simulink model "Controladoresplot"  (R2023b)
settings: Solver=ode1  StartTime=0.0  StopTime=70  FixedStep=1e-1  RelTol=1e-3  EnableMultiTasking=on
values from neighbouring files (symbols this model uses):
  C50_1 = 6.33    [P1.m]
  C50_2 = 6.76    [P2.m]
  C50_3 = 8.44    [P3.m]
  C50_4 = 6.44    [P4.m]
  Emax_1 = 94.1    [P1.m]
  Emax_2 = 86.0    (= 86)    [P2.m]
  Emax_3 = 80.7    [P3.m]
  Emax_4 = 102    [P4.m]
  gamma_1 = 2.24    [P1.m]
  gamma_2 = 4.29    [P2.m]
  gamma_3 = 4.10    (= 4.1)    [P3.m]
  gamma_4 = 2.18    [P4.m]
  k10_1 = Cl1_1 / V1    (= 0.38895787371)    [P1.m]
  k10_2 = Cl1_2 / V1    (= 0.37754352967)    [P2.m]
  k10_3 = Cl1_3 / V1    (= 0.386157411043)    [P3.m]
  k10_4 = Cl1_4 / V1    (= 0.323607493475)    [P4.m]
  k12_1 = Cl2_1 / V1    (= 0.375175644028)    [P1.m]
  k12_2 = Cl2_2 / V1    (= 0.397658079625)    [P2.m]
  k12_3 = Cl2_3 / V1    (= 0.44262295082)    [P3.m]
  k12_4 = Cl2_4 / V1    (= 0.318969555035)    [P4.m]
  k13_1 = Cl3_1 / V1    (= 0.195784543326)    [P1.m]
  k13_2 = Cl3_2 / V1    (= 0.195784543326)    [P2.m]
  k13_3 = Cl3_3 / V1    (= 0.195784543326)    [P3.m]
  k13_4 = Cl3_4 / V1    (= 0.195784543326)    [P4.m]
  k21_1 = Cl2_1/V2    (= 0.0667973147646)    [P1.m]
  k21_2 = Cl2_2/V2    (= 0.0664657298313)    [P2.m]
  k21_3 = Cl2_3/V2    (= 0.0659110723627)    [P3.m]
  k21_4 = Cl2_4/V2    (= 0.0678523389628)    [P4.m]
  k31_1 = Cl3_1/V3    (= 0.00351260504202)    [P1.m]
  k31_2 = Cl3_2/V3    (= 0.00351260504202)    [P2.m]
  k31_3 = Cl3_3/V3    (= 0.00351260504202)    [P3.m]
  k31_4 = Cl3_4/V3    (= 0.00351260504202)    [P4.m]
settings Model: Creator=Ana Gaby  LastModifiedBy=jeaze
settings SolverCC: AlgebraicLoopSolver=LineSearch
settings DataIOCC: LimitDataPoints=on  SaveFormat=Array  SignalLoggingSaveFormat=ModelDataLogs  ReturnWorkspaceOutputs=off
settings OptimizationCC: ExpressionDepthLimit=2147483647  LifeSpan=inf
settings DebuggingCC: UnderspecifiedInitializationDetection=Classic  MergeDetectMultiDrivingBlocksExec=none  SolverPrmCheckMsg=warning  FcnCallInpInsideContextMsg=warning  UnconnectedInputMsg=warning  UnconnectedOutputMsg=warning  UnconnectedLineMsg=warning  StateNameClashWarn=warning  SFUnexpectedBacktrackingDiag=warning  SFNoUnconditionalDefaultTransitionDiag=warning  SFExecutionAtInitializationDiag=none  ArithmeticOperatorsInVariantConditions=warning
settings HardwareCC: ProdBitPerPointer=32  ProdBitPerSizeT=32  ProdBitPerPtrDiffT=32  ProdLargestAtomicFloat=None  ProdIntDivRoundTo=Undefined  ProdEndianess=Unspecified  ProdWordSize=32  ProdHWDeviceType=32-bit Generic
settings ModelReferenceCC: EnableRefExpFcnMdlSchedulingChecks=on  PropagateSignalLabelsOutOfModel=off
settings SFSimCC: SimUseLocalCustomCode=off  SimParseCustomCode=off  CustomCodeUndefinedFunction=UseInterfaceOnly
settings RTWCC: RTWUseLocalCustomCode=off
settings CodeAppCC: StateflowObjectComments=on
settings GRTTargetCC: TargetLangStandard=C89/C90 (ANSI)  CombineOutputUpdateFcns=off  GRTInterface=on
settings ConfigComp: CovMetricSettings=dw  CovSaveCumulativeToWorkspaceVar=on  CovSaveSingleToWorkspaceVar=on  CovExternalEMLEnable=off

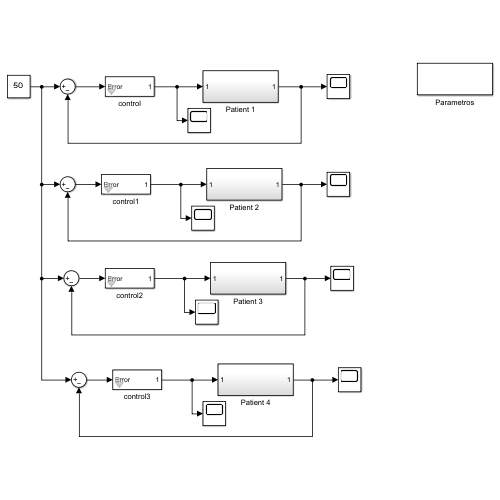
[thumbnail: Simulink's stored preview of the top-level diagram]
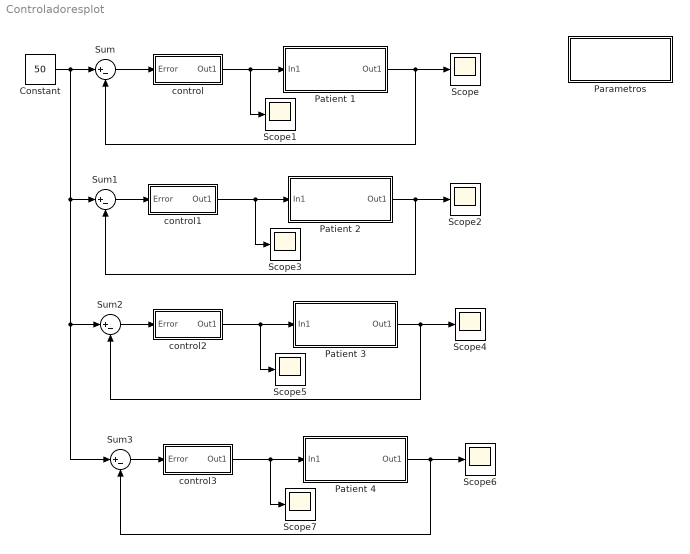
== system Controladoresplot ==
  Constant : Constant  Value=50
  Parametros : Subsystem
      settings: OpenFcn=|
      | P1
      | P2
      | P3
      | P4
  Patient 1 : Subsystem
  Patient 2 : Subsystem
  Patient 3 : Subsystem
  Patient 4 : Subsystem
  Scope{,1..7} (8 alike) : Scope
  Sum{,1..3} (4 alike) : Sum  Inputs=|+-
  control : Subsystem  mask{alfa=-100, Beta1=1}
  control1 : Subsystem  mask{alfa=-100, Beta1=1}
  control2 : Subsystem  mask{alfa=-100, Beta1=1}
  control3 : Subsystem  mask{alfa=-100, Beta1=1}
  wires:
  Patient 1/1(Out1) -> Scope/1, Sum/2
  control/1(Out1) -> Scope1/1, Patient 1/1(In1)
  Sum/1 -> control/1(Error)
  Constant/1 -> Sum/1, Sum1/1, Sum2/1, Sum3/1
  Patient 2/1(Out1) -> Scope2/1, Sum1/2
  control1/1(Out1) -> Patient 2/1(In1), Scope3/1
  Sum1/1 -> control1/1(Error)
  Patient 3/1(Out1) -> Scope4/1, Sum2/2
  control2/1(Out1) -> Patient 3/1(In1), Scope5/1
  Sum2/1 -> control2/1(Error)
  Patient 4/1(Out1) -> Scope6/1, Sum3/2
  control3/1(Out1) -> Patient 4/1(In1), Scope7/1
  Sum3/1 -> control3/1(Error)

== system Controladoresplot/Parametros ==

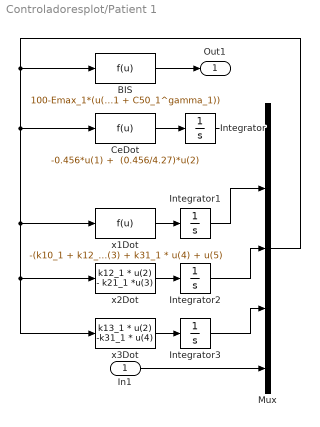
== system Controladoresplot/Patient 1 ==
  In1 : Inport
  BIS : Fcn  Expr=100-Emax_1*(u(1)^gamma_1/(u(1)^gamma_1 + C50_1^gamma_1))
  CeDot : Fcn  Expr="-0.456*u(1) +  (0.456/4.27)*u(2)"
  Integrator{,1..3} (4 alike) : Integrator
  Mux : Mux  Inputs=5
  x1Dot : Fcn  Expr=-(k10_1 + k12_1 + k13_1)*u(2) + k21_1 * u(3) + k31_1 * u(4) + u(5)
  x2Dot : Fcn  Expr=k12_1 * u(2) - k21_1 *u(3)
  x3Dot : Fcn  Expr=k13_1 * u(2) -k31_1 * u(4)
  Out1 : Outport  VectorParamsAs1DForOutWhenUnconnected=off
  wires:
  BIS/1 -> Out1/1
  CeDot/1 -> Integrator/1
  x1Dot/1 -> Integrator1/1
  x2Dot/1 -> Integrator2/1
  x3Dot/1 -> Integrator3/1
  Integrator/1 -> Mux/1
  Integrator1/1 -> Mux/2
  Integrator2/1 -> Mux/3
  Integrator3/1 -> Mux/4
  In1/1 -> Mux/5
  Mux/1 -> x3Dot/1, x2Dot/1, x1Dot/1, CeDot/1, BIS/1

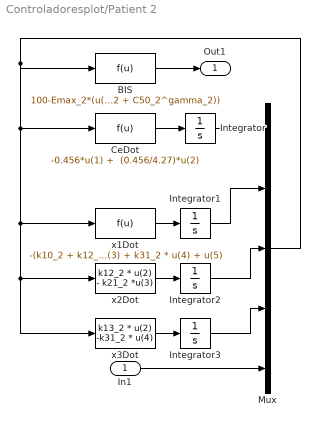
== system Controladoresplot/Patient 2 ==
  In1 : Inport
  BIS : Fcn  Expr=100-Emax_2*(u(1)^gamma_2/(u(1)^gamma_2 + C50_2^gamma_2))
  CeDot : Fcn  Expr="-0.456*u(1) +  (0.456/4.27)*u(2)"
  Integrator{,1..3} (4 alike) : Integrator
  Mux : Mux  Inputs=5
  x1Dot : Fcn  Expr=-(k10_2 + k12_2 + k13_2)*u(2) + k21_2 * u(3) + k31_2 * u(4) + u(5)
  x2Dot : Fcn  Expr=k12_2 * u(2) - k21_2 *u(3)
  x3Dot : Fcn  Expr=k13_2 * u(2) -k31_2 * u(4)
  Out1 : Outport  VectorParamsAs1DForOutWhenUnconnected=off
  wires:
  BIS/1 -> Out1/1
  CeDot/1 -> Integrator/1
  x1Dot/1 -> Integrator1/1
  x2Dot/1 -> Integrator2/1
  x3Dot/1 -> Integrator3/1
  Integrator/1 -> Mux/1
  Integrator1/1 -> Mux/2
  Integrator2/1 -> Mux/3
  Integrator3/1 -> Mux/4
  In1/1 -> Mux/5
  Mux/1 -> x3Dot/1, x2Dot/1, x1Dot/1, CeDot/1, BIS/1

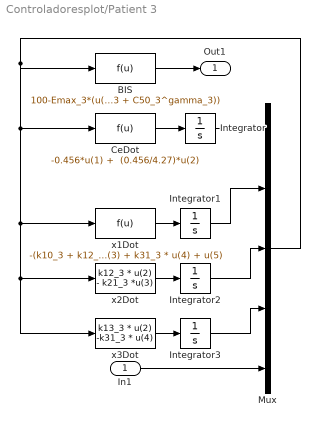
== system Controladoresplot/Patient 3 ==
  In1 : Inport
  BIS : Fcn  Expr=100-Emax_3*(u(1)^gamma_3/(u(1)^gamma_3 + C50_3^gamma_3))
  CeDot : Fcn  Expr="-0.456*u(1) +  (0.456/4.27)*u(2)"
  Integrator{,1..3} (4 alike) : Integrator
  Mux : Mux  Inputs=5
  x1Dot : Fcn  Expr=-(k10_3 + k12_3 + k13_3)*u(2) + k21_3 * u(3) + k31_3 * u(4) + u(5)
  x2Dot : Fcn  Expr=k12_3 * u(2) - k21_3 *u(3)
  x3Dot : Fcn  Expr=k13_3 * u(2) -k31_3 * u(4)
  Out1 : Outport  VectorParamsAs1DForOutWhenUnconnected=off
  wires:
  BIS/1 -> Out1/1
  CeDot/1 -> Integrator/1
  x1Dot/1 -> Integrator1/1
  x2Dot/1 -> Integrator2/1
  x3Dot/1 -> Integrator3/1
  Integrator/1 -> Mux/1
  Integrator1/1 -> Mux/2
  Integrator2/1 -> Mux/3
  Integrator3/1 -> Mux/4
  In1/1 -> Mux/5
  Mux/1 -> x3Dot/1, x2Dot/1, x1Dot/1, CeDot/1, BIS/1

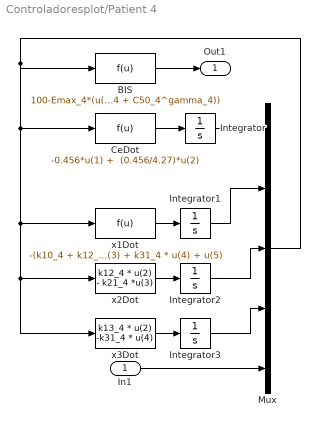
== system Controladoresplot/Patient 4 ==
  In1 : Inport
  BIS : Fcn  Expr=100-Emax_4*(u(1)^gamma_4/(u(1)^gamma_4 + C50_4^gamma_4))
  CeDot : Fcn  Expr="-0.456*u(1) +  (0.456/4.27)*u(2)"
  Integrator{,1..3} (4 alike) : Integrator
  Mux : Mux  Inputs=5
  x1Dot : Fcn  Expr=-(k10_4 + k12_4 + k13_4)*u(2) + k21_4 * u(3) + k31_4 * u(4) + u(5)
  x2Dot : Fcn  Expr=k12_4 * u(2) - k21_4 *u(3)
  x3Dot : Fcn  Expr=k13_4 * u(2) -k31_4 * u(4)
  Out1 : Outport  VectorParamsAs1DForOutWhenUnconnected=off
  wires:
  BIS/1 -> Out1/1
  CeDot/1 -> Integrator/1
  x1Dot/1 -> Integrator1/1
  x2Dot/1 -> Integrator2/1
  x3Dot/1 -> Integrator3/1
  Integrator/1 -> Mux/1
  Integrator1/1 -> Mux/2
  Integrator2/1 -> Mux/3
  Integrator3/1 -> Mux/4
  In1/1 -> Mux/5
  Mux/1 -> x3Dot/1, x2Dot/1, x1Dot/1, CeDot/1, BIS/1

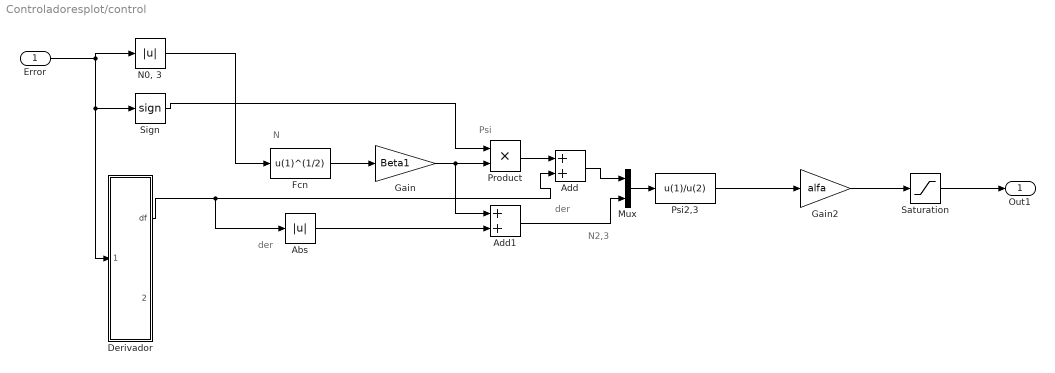
== system Controladoresplot/control ==
  note: Psi
  note: N
  note: der
  note: der
  note: N2,3
  Error : Inport
  Abs : Abs  SaturateOnIntegerOverflow=off
  Add : Sum
  Add1 : Sum
  Derivador : Subsystem
  Fcn : Fcn  Expr=u(1)^(1/2)
  Gain : Gain  Gain=Beta1
  Gain2 : Gain  Gain=alfa
  Mux : Mux  Inputs=2
  "N0, 3" : Abs  SaturateOnIntegerOverflow=off
  Product : Product  RndMeth=Zero
  Psi2,3 : Fcn  Expr=u(1)/u(2)
  Saturation : Saturate  UpperLimit=inf  LowerLimit=0
  Sign : Signum
  Out1 : Outport  VectorParamsAs1DForOutWhenUnconnected=off
  wires:
  Error/1 -> "N0, 3"/1, Sign/1, Derivador/1(In1)
  Fcn/1 -> Gain/1
  Gain/1 -> Product/2, Add1/1
  Product/1 -> Add/1
  Abs/1 -> Add1/2
  Mux/1 -> Psi2,3/1
  Add/1 -> Mux/1
  Add1/1 -> Mux/2
  "N0, 3"/1 -> Fcn/1
  Sign/1 -> Product/1
  Derivador/1(df) -> Abs/1, Add/2
  Gain2/1 -> Saturation/1
  Saturation/1 -> Out1/1
  Psi2,3/1 -> Gain2/1

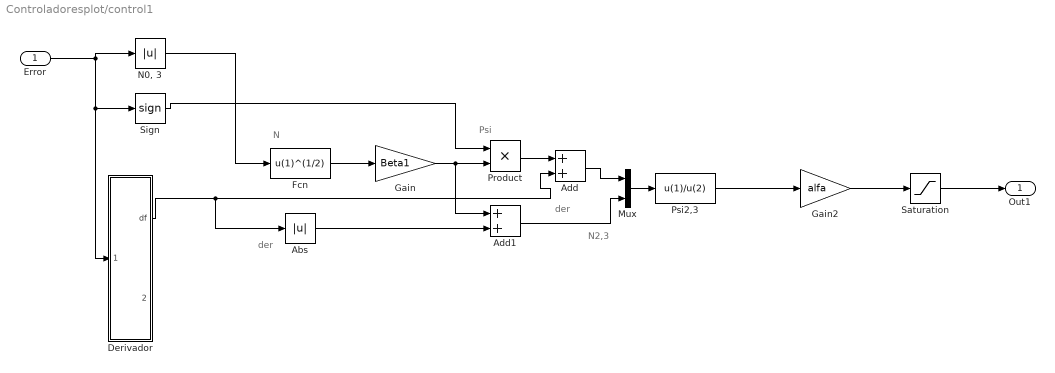
== system Controladoresplot/control1 ==
  note: Psi
  note: N
  note: der
  note: der
  note: N2,3
  Error : Inport
  Abs : Abs  SaturateOnIntegerOverflow=off
  Add : Sum
  Add1 : Sum
  Derivador : Subsystem
  Fcn : Fcn  Expr=u(1)^(1/2)
  Gain : Gain  Gain=Beta1
  Gain2 : Gain  Gain=alfa
  Mux : Mux  Inputs=2
  "N0, 3" : Abs  SaturateOnIntegerOverflow=off
  Product : Product  RndMeth=Zero
  Psi2,3 : Fcn  Expr=u(1)/u(2)
  Saturation : Saturate  UpperLimit=inf  LowerLimit=0
  Sign : Signum
  Out1 : Outport  VectorParamsAs1DForOutWhenUnconnected=off
  wires:
  Error/1 -> "N0, 3"/1, Sign/1, Derivador/1(In1)
  Fcn/1 -> Gain/1
  Gain/1 -> Product/2, Add1/1
  Product/1 -> Add/1
  Abs/1 -> Add1/2
  Mux/1 -> Psi2,3/1
  Add/1 -> Mux/1
  Add1/1 -> Mux/2
  "N0, 3"/1 -> Fcn/1
  Sign/1 -> Product/1
  Derivador/1(df) -> Abs/1, Add/2
  Gain2/1 -> Saturation/1
  Saturation/1 -> Out1/1
  Psi2,3/1 -> Gain2/1

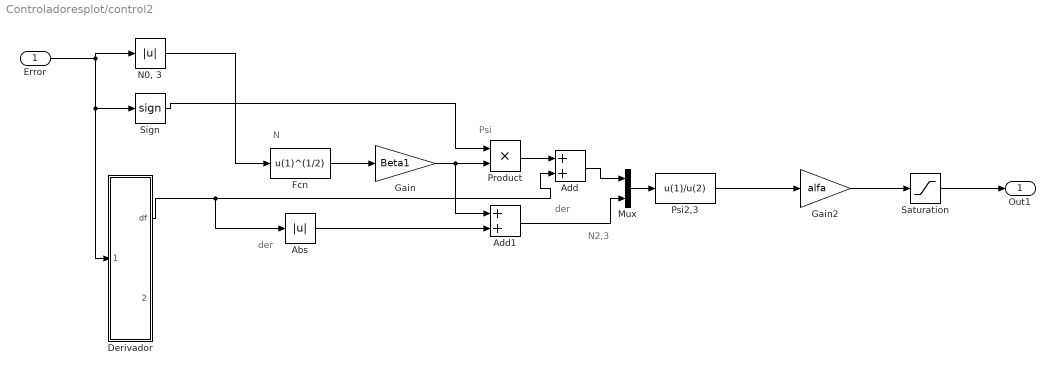
== system Controladoresplot/control2 ==
  note: Psi
  note: N
  note: der
  note: der
  note: N2,3
  Error : Inport
  Abs : Abs  SaturateOnIntegerOverflow=off
  Add : Sum
  Add1 : Sum
  Derivador : Subsystem
  Fcn : Fcn  Expr=u(1)^(1/2)
  Gain : Gain  Gain=Beta1
  Gain2 : Gain  Gain=alfa
  Mux : Mux  Inputs=2
  "N0, 3" : Abs  SaturateOnIntegerOverflow=off
  Product : Product  RndMeth=Zero
  Psi2,3 : Fcn  Expr=u(1)/u(2)
  Saturation : Saturate  UpperLimit=inf  LowerLimit=0
  Sign : Signum
  Out1 : Outport  VectorParamsAs1DForOutWhenUnconnected=off
  wires:
  Error/1 -> "N0, 3"/1, Sign/1, Derivador/1(In1)
  Fcn/1 -> Gain/1
  Gain/1 -> Product/2, Add1/1
  Product/1 -> Add/1
  Abs/1 -> Add1/2
  Mux/1 -> Psi2,3/1
  Add/1 -> Mux/1
  Add1/1 -> Mux/2
  "N0, 3"/1 -> Fcn/1
  Sign/1 -> Product/1
  Derivador/1(df) -> Abs/1, Add/2
  Gain2/1 -> Saturation/1
  Saturation/1 -> Out1/1
  Psi2,3/1 -> Gain2/1

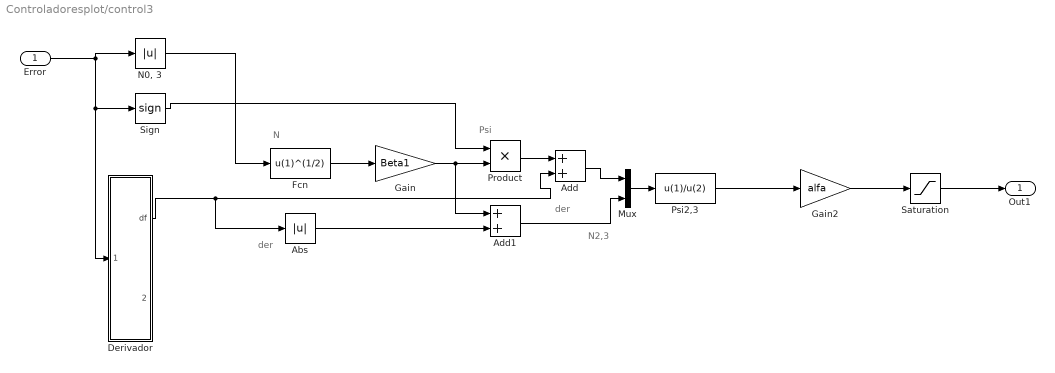
== system Controladoresplot/control3 ==
  note: Psi
  note: N
  note: der
  note: der
  note: N2,3
  Error : Inport
  Abs : Abs  SaturateOnIntegerOverflow=off
  Add : Sum
  Add1 : Sum
  Derivador : Subsystem
  Fcn : Fcn  Expr=u(1)^(1/2)
  Gain : Gain  Gain=Beta1
  Gain2 : Gain  Gain=alfa
  Mux : Mux  Inputs=2
  "N0, 3" : Abs  SaturateOnIntegerOverflow=off
  Product : Product  RndMeth=Zero
  Psi2,3 : Fcn  Expr=u(1)/u(2)
  Saturation : Saturate  UpperLimit=inf  LowerLimit=0
  Sign : Signum
  Out1 : Outport  VectorParamsAs1DForOutWhenUnconnected=off
  wires:
  Error/1 -> "N0, 3"/1, Sign/1, Derivador/1(In1)
  Fcn/1 -> Gain/1
  Gain/1 -> Product/2, Add1/1
  Product/1 -> Add/1
  Abs/1 -> Add1/2
  Mux/1 -> Psi2,3/1
  Add/1 -> Mux/1
  Add1/1 -> Mux/2
  "N0, 3"/1 -> Fcn/1
  Sign/1 -> Product/1
  Derivador/1(df) -> Abs/1, Add/2
  Gain2/1 -> Saturation/1
  Saturation/1 -> Out1/1
  Psi2,3/1 -> Gain2/1

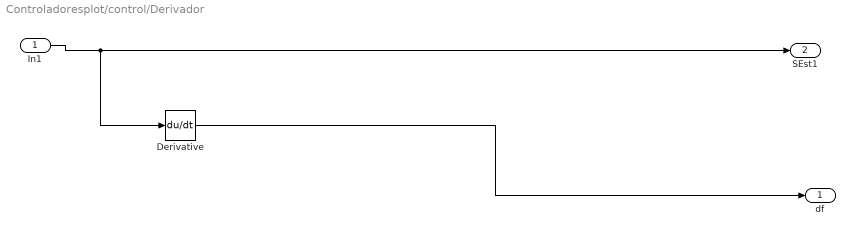
== system Controladoresplot/control/Derivador ==
  In1 : Inport
  Derivative : Derivative
  df : Outport  VectorParamsAs1DForOutWhenUnconnected=off
  SEst1 : Outport  Port=2  VectorParamsAs1DForOutWhenUnconnected=off
  wires:
  In1/1 -> Derivative/1, SEst1/1
  Derivative/1 -> df/1

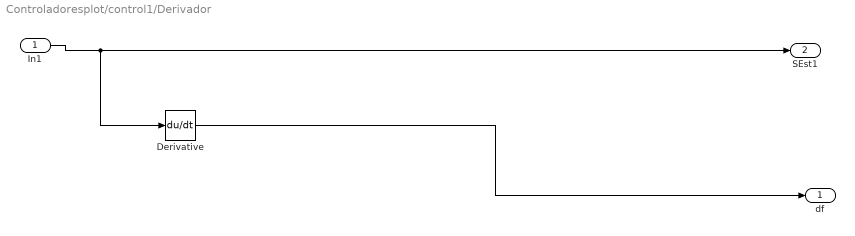
== system Controladoresplot/control1/Derivador ==
  In1 : Inport
  Derivative : Derivative
  df : Outport  VectorParamsAs1DForOutWhenUnconnected=off
  SEst1 : Outport  Port=2  VectorParamsAs1DForOutWhenUnconnected=off
  wires:
  In1/1 -> Derivative/1, SEst1/1
  Derivative/1 -> df/1

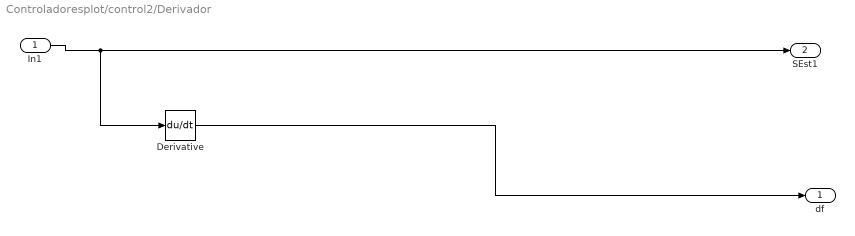
== system Controladoresplot/control2/Derivador ==
  In1 : Inport
  Derivative : Derivative
  df : Outport  VectorParamsAs1DForOutWhenUnconnected=off
  SEst1 : Outport  Port=2  VectorParamsAs1DForOutWhenUnconnected=off
  wires:
  In1/1 -> Derivative/1, SEst1/1
  Derivative/1 -> df/1

== system Controladoresplot/control3/Derivador ==
  In1 : Inport
  Derivative : Derivative
  df : Outport  VectorParamsAs1DForOutWhenUnconnected=off
  SEst1 : Outport  Port=2  VectorParamsAs1DForOutWhenUnconnected=off
  wires:
  In1/1 -> Derivative/1, SEst1/1
  Derivative/1 -> df/1
